simulink model "HW03_Tirel_Sim1_MIMO"  (R2020b)
settings: Solver=VariableStepAuto  StartTime=0.0  StopTime=20  RelTol=1e-3
undefined symbols (not defined in the file or in its folder): K
libraries: cstblocks x2
settings Model: Creator=DELL  LastModifiedBy=DELL

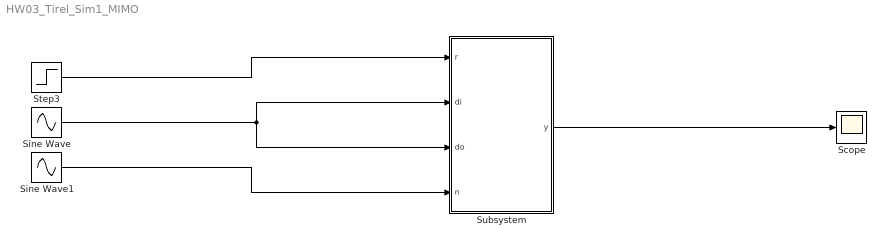
== system HW03_Tirel_Sim1_MIMO ==
  Scope : Scope
  Sine Wave : Sin  Frequency=5  SampleTime=0
  Sine Wave1 : Sin  Frequency=500  SampleTime=0
  Step3 : Step  Time=0  After=10  SampleTime=0
  Subsystem : Subsystem
  wires:
  Sine Wave/1 -> Subsystem/2(di), Subsystem/3(do)
  Sine Wave1/1 -> Subsystem/4(n)
  Step3/1 -> Subsystem/1(r)
  Subsystem/1(y) -> Scope/1

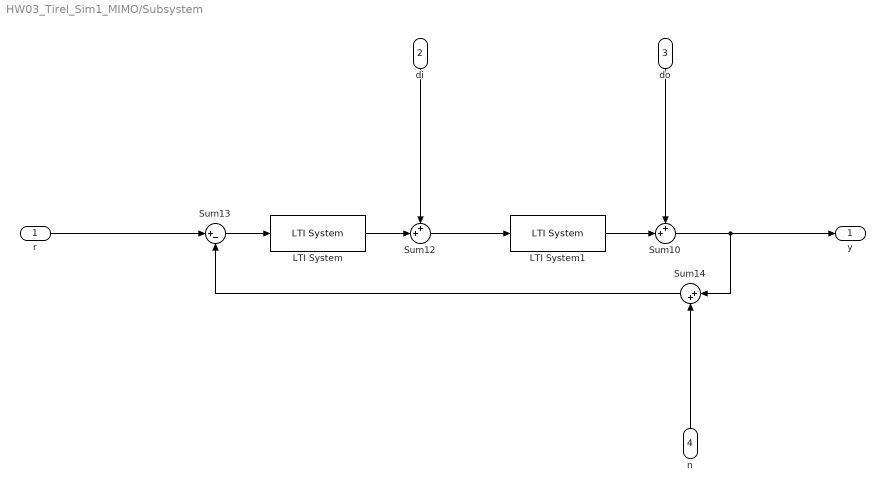
== system HW03_Tirel_Sim1_MIMO/Subsystem ==
  r : Inport
  di : Inport  Port=2
  do : Inport  Port=3
  n : Inport  Port=4
  LTI System : cstblocks/LTI System  sys=tf(K)  IC=[]
  LTI System1 : cstblocks/LTI System  sys=W  IC=[]
  Sum10 : Sum  Inputs=++|
  Sum12 : Sum  Inputs=++|
  Sum13 : Sum  Inputs=|+-
  Sum14 : Sum  Inputs=|++
  y : Outport
  wires:
  Sum10/1 -> y/1, Sum14/1
  Sum12/1 -> LTI System1/1
  Sum14/1 -> Sum13/2
  di/1 -> Sum12/1
  Sum13/1 -> LTI System/1
  r/1 -> Sum13/1
  do/1 -> Sum10/1
  n/1 -> Sum14/2
  LTI System1/1 -> Sum10/2
  LTI System/1 -> Sum12/2
